simulink model "Fuzzy1_Calculate_output_values"  (R2017b)
settings: Solver=VariableStepAuto  StartTime=0.0  StopTime=100.0  RelTol=1e-3
libraries: fuzblock x1
settings Model: Creator=me  LastModifiedBy=me

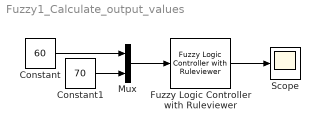
== system Fuzzy1_Calculate_output_values ==
  Constant : Constant  Value=60
  Constant1 : Constant  Value=70
  Fuzzy Logic Controller with Ruleviewer : fuzblock/Fuzzy Logic  Controller  with Ruleviewer  fismatrix=Fuzzy  Ts=2
  Mux : Mux  Inputs=2
  Scope : Scope
  wires:
  Mux/1 -> Fuzzy Logic Controller with Ruleviewer/1
  Constant/1 -> Mux/1
  Constant1/1 -> Mux/2
  Fuzzy Logic Controller with Ruleviewer/1 -> Scope/1
